simulink subsystem "CANOutputs"  (R2022b)
settings: Solver=VariableStepAuto  StartTime=0.0  StopTime=10.0  RelTol=1e-3
settings Model: Creator=serga  LastModifiedBy=serga

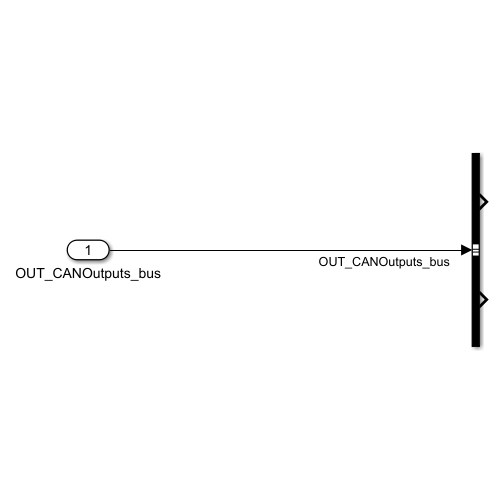
[thumbnail: Simulink's stored preview of the top-level diagram]
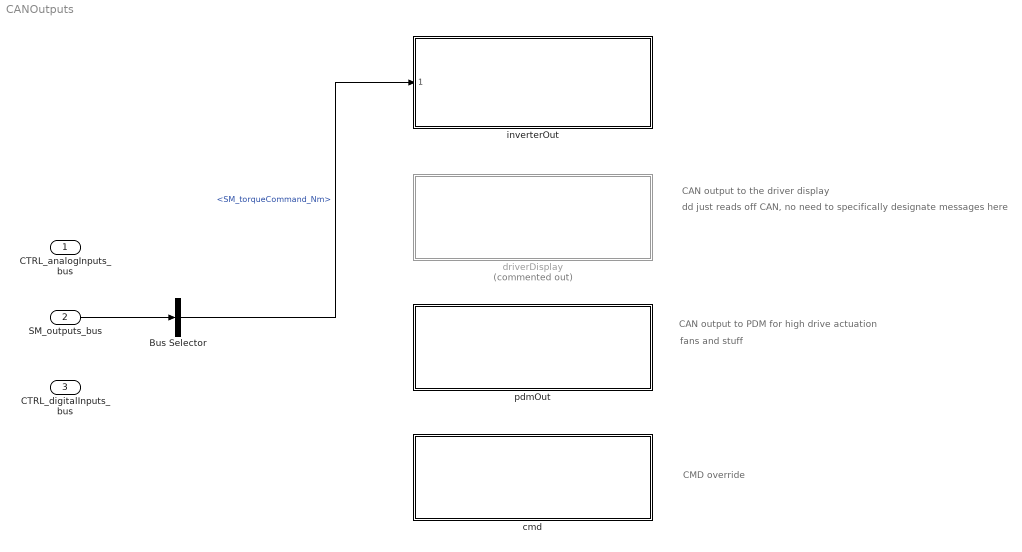
== system CANOutputs ==
  note: fans and stuff
  note: dd just reads off CAN, no need to specifically designate messages here
  note: CMD override
  note: CAN output to PDM for high drive actuation
  note: CAN output to the driver display
  CTRL_analogInputs_bus : Inport
  SM_outputs_bus : Inport  Port=2
  CTRL_digitalInputs_bus : Inport  Port=3
  Bus Selector : BusSelector  OutputSignals=SM_tractive_bus.SM_torqueCommand_Nm
  cmd : Subsystem  ReferencedSubsystem=cmd
  driverDisplay : Subsystem  Commented=on  ReferencedSubsystem=driverDisplay
  inverterOut : Subsystem  ReferencedSubsystem=inverterOut
  pdmOut : Subsystem  ReferencedSubsystem=pdmOut
  wires:
  SM_outputs_bus/1 -> Bus Selector/1
  Bus Selector/1 -> inverterOut/1  "<SM_torqueCommand_Nm>"
